simulink model "Ball_and_Plate_MicroLabBox_student_v2019"  (R2019b)
settings: Solver=ode1  StartTime=0.0  StopTime=Inf  FixedStep=0.001  RelTol=1e-3
PostLoadFcn:
  | , if any(exist('dsrtsu_mdlpostloadfcn', 'file') ~= 0), dsrtsu_mdlpostloadfcn('Execute', bdroot); end,
InitFcn:
  | , if any(exist('rtifpga_mdlclblib', 'file') ~= 0), rtifpga_mdlclblib('Init', bdroot); end,
values from neighbouring files (symbols this model uses):
  A_robust = K_robust.A    [Init_workspace.m]    (also in OptimalControlleerSythesisNew.m = K.A)
  B_robust = K_robust.B    [Init_workspace.m]    (also in OptimalControlleerSythesisNew.m = K.B)
  ball_pos_sat = 0.2    [Init_workspace.m]
  ball_vel_sat = 1    [Init_workspace.m]
  Baw_robust = C_robust' / (C_robust*C_robust' + aw_reg*eye(2))    [OptimalControlleerSythesisNew.m]
  C_robust = K_robust.C    [Init_workspace.m]    (also in OptimalControlleerSythesisNew.m = K.C)
  D_robust = K_robust.D    [Init_workspace.m]    (also in OptimalControlleerSythesisNew.m = K.D)
  g = 9.81    [Init_workspace.m]    (also in OptimalControlleerSythesis.m; OptimalControlleerSythesisNew.m; Robustcontroller_angleOutput_Hinf_positionSensitive_center034.m; compute_mpc_params.m)
  K_lqr = dlqr(Ad, Bd, Q_lqr, R_lqr)    [Init_workspace.m]
  Kaw_robust = 0.15    [OptimalControlleerSythesisNew.m]
  path = quintic(-0.0289,3,0,1/fs)    [Init_workspace.m]    (also in Quintic_Time.m = reference_end; Quintic_Velocity.m = reference_end)
  plate_angle_sat = deg2rad(10)    [Init_workspace.m]
  Q_kf = diag([1, 100, 1, 100])    [Init_workspace.m]
  R_kf = diag([0.1, 0.1])    [Init_workspace.m]
  Ts_Outer = 1/50    (= 0.02)    [Init_workspace.m]
  u_max_robust = [ alpha_lim;  beta_lim]    [OptimalControlleerSythesisNew.m]
  u_min_robust = [-alpha_lim; -beta_lim]    [OptimalControlleerSythesisNew.m]
  uA = repmat(uA,[1,P])    [Init_workspace.m]
  uB = repmat(uB,[1,P])    [Init_workspace.m]
  uC = repmat(uC,[1,P])    [Init_workspace.m]
undefined symbols (not defined in the file or in its folder): a_circ, a_square, DiscIntNeverNeededParam, inner_I_sat, r_circ, r_square, Ts_Inner
libraries: simulink x7, rtiemclib x6, rtiethernetlib x3, rti1202lib_dac_class1 x3, slrealtimeutilitieslib x1, mpclib x1
(part 3 of 3)

== system Ball_and_Plate_MicroLabBox_student_v2019/Innerloop_Actuator/Motor_C/Position Measurement ==
  Init : Inport
  AbsPosition : Sum  Inputs=-+-  SaturateOnIntegerOverflow=on
  Constant : Constant  Value=10
  EMC_ENCODER_BL1 : rtiemclib/EMC_ENCODER_BL1  DSProperties=struct('RTI',struct('Version',uint32(2),'BlockType',struct('isSLSource',uint8(1),'isSLSink',uint8(0),'isHWSource',uint8(1),'isHWSink',uint8(0),'isSetup',uint8(0),'isInline',uint8(1),'isNonInline',uint8(0),'isInterrupt',uint8(0),'isChannelwise',uint8(1)),'IOBoardType','DSEMC','UnitType','ENCODER','Identifier','ENCODER','DialogType','ML','BlockSet','RTIEMC','SlaveProcessor','NONE'))  RTIBlockInterface=struct('OutputPortsWidth',int32([1 1 1]),'OutputPortsActive',int32([1 1 0]),'OutputPortsName',{{'Position','Speed',['Index Detected']}},'OutputPortsDataType',{{'SS_DOUBLE','SS_DOUBLE','SS_BOOLEAN'}},'InitLevel',3,'IconTransparency','on','BlockDisplay',{{['EMC Encoder\nUnit: 3\nDIO class: 2\nPort: 1\nChannel: 5'],'center'}},'DialogFcn','rtiemcencodergui','BlockName',struct('Token',{{'EMC_ENCODER_BL1'}}))  RTIBlockParameters=struct('UnitNo',{{3,'OFF',[1 6]}},'DioClassNo',{{2,'OFF',[1 2]}},'PortNo',{{1,'OFF',[1 1]}},'ChannelNo',{{5,'OFF',[1 11]}},'HwSignalPin',{{['DIO1 ch1'],'OFF',[]}},'HwRefPin',{{'GND','OFF',[]}},'EnablePosMeasurement',{{1,'OFF',[0 1]}},'IndexSetMode',{{1,'OFF',[1 3]}},'EnableMinSpeed',{{0,'OFF',[0 1]}},'NumOfLines',{{'1024','OFF',[1 2097152]}},'InitAngleValue',{{'60','OFF',[0 359.99999]}},'IndexAngleValue',{{'0','OFF',[0 359.99999]}},'MinSpeedAngleValue',{{'45','OFF',[0.05 10000]}},'MinPosValue',{{'0','OFF',[-2097152 2097150.75]}},'MaxPosValue',{{'10000','OFF',[-2097151 2097151.75]}},'InitPosValue',{{'0','OFF',[-2097152 2097151.75]}},'IndexPosValue',{{'0','OFF',[-2097152 2097151.75]}},'MinSpeedPosValue',{{'100','OFF',[1 1000000]}},'IndexGateMode',{{0,'OFF',[0 1]}},'EnableNoiseFilter',{{0,'OFF',[0 1]}},'FilterInterval',{{'0','OFF',[0 0.01]}},'IndexDetectedOutPortMode',{{0,'OFF',[0 1]}},'BuildCheckAngleMeasurement',{{0,'OFF',[0 1]}},'BuildCheckAngleIndexMode',{{0,'OFF',[0 1]}},'BuildCheckPosIndexMode',{{0,'OFF',[0 1]}},'BuildCheckAngleMinSpeed',{{0,'OFF',[0 1]}},'BuildCheckPosMinSpeed',{{0,'OFF',[0 1]}},'TLCFileName',{{'rtiemcencoder','OFF',[]}})  RTISFcnParameters=struct('UnitNo','int32','DioClassNo','int32','PortNo','int32','ChannelNo','int32','EnablePosMeasurement','int32','IndexSetMode','int32','IndexDetectedOutPortMode','int32','EnableMinSpeed','int32','NumOfLines','uint32','InitAngleValue','double','IndexAngleValue','double','MinSpeedAngleValue','double','MinPosValue','double','MaxPosValue','double','InitPosValue','double','IndexPosValue','double','MinSpeedPosValue','double','IndexGateMode','int32','EnableNoiseFilter','int32','FilterInterval','double','TLCFileName','char')  RTIBlockParaDefault=struct('UnitNo',1,'DioClassNo',1,'PortNo',1,'ChannelNo',1,'HwSignalPin',['DIO1 ch1'],'HwRefPin','GND','EnablePosMeasurement',0,'IndexSetMode',1,'EnableMinSpeed',0,'NumOfLines',1024,'InitAngleValue',60,'IndexAngleValue',0,'MinSpeedAngleValue',45,'MinPosValue',0,'MaxPosValue',1023.75,'InitPosValue',0,'IndexPosValue',0,'MinSpeedPosValue',100,'IndexGateMode',0,'EnableNoiseFilter',0,'FilterInterval',0,'IndexDetectedOutPortMode',0,'BuildCheckAngleMeasurement',1,'BuildCheckAngleIndexMode',0,'BuildCheckPosIndexMode',0,'BuildCheckAngleMinSpeed',0,'BuildCheckPosMinSpeed',0,'TLCFileName','rtiemcencoder')
      settings: SourceProductName=dSPACE RTI Electric Motor Control Blockset
  EMC_ENCODER_POS_SET_BL1 : rtiemclib/EMC_ENCODER_POS_SET_BL1  DSProperties=struct('RTI',struct('Version',uint32(1),'BlockType',struct('isSLSource',uint8(0),'isSLSink',uint8(1),'isHWSource',uint8(0),'isHWSink',uint8(1),'isSetup',uint8(0),'isInline',uint8(1),'isNonInline',uint8(0),'isInterrupt',uint8(0),'isChannelwise',uint8(1)),'IOBoardType','DSEMC','UnitType','ENCODER','Identifier','ENCODERPOSSET','DialogType','ML','BlockSet','RTIEMC','SlaveProcessor','NONE'))  RTIBlockInterface=struct('InputPortsWidth',int32(1),'InputPortsActive',1,'InputPortsDataType',{{'SS_DOUBLE'}},'InputPortsName',{{'Position'}},'TriggerPort',{{'rising'}},'InitLevel',3,'IconTransparency','on','BlockDisplay',{{['EMC Encoder Position Set\nUnit: 3\nDIO class: 2\nPort: 1\nChannel: 5'],'center'}},'DialogFcn','rtiemcencoderpossetgui','BlockName',struct('Token',{{'EMC_ENCODER_POS_SET_BL1'}}))  RTIBlockParameters=struct('EncoderIdIndex',{{4,'OFF',[1 4]}},'UnitNo',{{3,'OFF',[]}},'DioClassNo',{{2,'OFF',[]}},'PortNo',{{1,'OFF',[]}},'ChannelNo',{{5,'OFF',[]}},'EnablePosMeasurement',{{1,'OFF',[]}},'NumOfLines',{{1024,'OFF',[]}},'TLCFileName',{{'rtiemcencoderposset','OFF',[]}})  RTISFcnParameters=struct('EncoderIdIndex','int32','UnitNo','int32','DioClassNo','int32','PortNo','int32','ChannelNo','int32','EnablePosMeasurement','int32','NumOfLines','int32','TLCFileName','char')  RTIBlockParaDefault=struct('EncoderIdIndex',1,'UnitNo',-1,'DioClassNo',-1,'PortNo',-1,'ChannelNo',-1,'EnablePosMeasurement',0,'NumOfLines',1024,'TLCFileName','rtiemcencoderposset')
      settings: SourceProductName=dSPACE RTI Electric Motor Control Blockset
  Inc2Pos : Gain  Gain=8e-3  SaturateOnIntegerOverflow=on  OutDataTypeStr=Inherit: Same as input  ParamDataTypeStr=Inherit: Same as input
  Initial : Subsystem
  Pos_offset : Constant  Value=0
  ZP : Constant  Value=29
  mm2m : Gain  Gain=0.001
  init_current : Outport  VectorParamsAs1DForOutWhenUnconnected=off
  Position [m] : Outport  Port=2  VectorParamsAs1DForOutWhenUnconnected=off
  wires:
  AbsPosition/1 -> mm2m/1
  Inc2Pos/1 -> Initial/1(Pos), AbsPosition/2
  Initial/2(init_current) -> init_current/1
  mm2m/1 -> Position [m]/1
  EMC_ENCODER_BL1/2 -> Initial/2(DeltaPos)
  ZP/1 -> AbsPosition/1
  Constant/1 -> EMC_ENCODER_POS_SET_BL1/1
  Init/1 -> Initial/3(Init), EMC_ENCODER_POS_SET_BL1/Trigger
  Pos_offset/1 -> AbsPosition/3
  EMC_ENCODER_BL1/1 -> Inc2Pos/1

== system Ball_and_Plate_MicroLabBox_student_v2019/Innerloop_Actuator/Motor_C/motorC ==
  Input : Inport
  I_reset : Inport  Port=2
  Add : Sum
  Dct1lowpass1 : S-Function  FunctionName=dlowpass1  Parameters=f_den, 0.001  SFunctionDeploymentMode=off  EnableBusSupport=off  mask(dctools){f_den=50}
      mask prompts: f_den "Pole [Hz]"
      mask help: This block implements a discrete time 1st order lowpass filter.
      mask Display: disp('DCT 1st order lowpass')
  Dct1lowpass2 : S-Function  Commented=on  FunctionName=dlowpass1  Parameters=f_den, 0.001  SFunctionDeploymentMode=off  EnableBusSupport=off  mask(dctools){f_den=50}
      mask prompts: f_den "Pole [Hz]"
      mask help: This block implements a discrete time 1st order lowpass filter.
      mask Display: disp('DCT 1st order lowpass')
  Dctleadlag1 : S-Function  FunctionName=dleadlag  Parameters=f_num, f_den, 0.001  SFunctionDeploymentMode=off  EnableBusSupport=off  mask(dctools){f_num=7.5, f_den=30}
      mask prompts: f_num "Zero [Hz]"; f_den "Pole [Hz]"
      mask help: This block implements a discrete time leadlag filter.
      mask Display: disp('DCT leadlag')
  Dctleadlag2 : S-Function  Commented=on  FunctionName=dleadlag  Parameters=f_num, f_den, 0.001  SFunctionDeploymentMode=off  EnableBusSupport=off  mask(dctools){f_num=7.5, f_den=45}
      mask prompts: f_num "Zero [Hz]"; f_den "Pole [Hz]"
      mask help: This block implements a discrete time leadlag filter.
      mask Display: disp('DCT leadlag')
  Discrete-Time Integrator : DiscreteIntegrator  gainval=2500  ExternalReset=rising  SampleTime=-1  LimitOutput=on  UpperSaturationLimit=inner_I_sat  LowerSaturationLimit=-inner_I_sat  ICPrevOutput=DiscIntNeverNeededParam  ICPrevScaledInput=DiscIntNeverNeededParam
  Gain1 : Gain  Commented=on  Gain=350  SaturateOnIntegerOverflow=on  OutDataTypeStr=Inherit: Same as input  ParamDataTypeStr=Inherit: Same as input
  Gain2 : Gain  Gain=400  SaturateOnIntegerOverflow=on  OutDataTypeStr=Inherit: Same as input  ParamDataTypeStr=Inherit: Same as input
  Output : Outport
  wires:
  Add/1 -> Output/1
  Dctleadlag1/1 -> Dct1lowpass1/1
  Input/1 -> Gain2/1, Discrete-Time Integrator/1
  Dct1lowpass1/1 -> Add/1
  I_reset/1 -> Discrete-Time Integrator/2
  Gain2/1 -> Dctleadlag1/1
  Discrete-Time Integrator/1 -> Add/2
  Gain1/1 -> Dctleadlag2/1
  Dctleadlag2/1 -> Dct1lowpass2/1

== system Ball_and_Plate_MicroLabBox_student_v2019/RTI Data/RTI Data Store/RTI Data Store ==
  RTI Data Store : Subsystem  mask(RTI_DATA_STORE){}
      mask help:
      | RTI Data Store Block. This block is used by RTI to store internal model dependent data. Deleting this block will result in data loss.
      |
      | NEVER DELETE, COPY, OR MODIFY THIS BLOCK!
      mask Help:
      | RTI Data Store Block. This block is used by RTI to store internal model dependent data. Deleting this block will result in data loss.
      | 
      | NEVER DELETE, COPY, OR MODIFY THIS BLOCK!
      mask Display: text(0.5, 0.5, ' ', 'HorizontalAlignment', 'center');

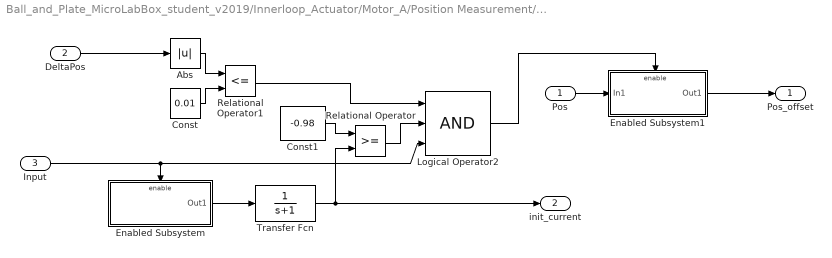
== system Ball_and_Plate_MicroLabBox_student_v2019/Innerloop_Actuator/Motor_A/Position Measurement/Initial ==
  Pos : Inport
  DeltaPos : Inport  Port=2
  Input : Inport  Port=3
  Abs : Abs  SaturateOnIntegerOverflow=on
  Const : Constant  Value=0.01
  Const1 : Constant  Value=-0.98
  Enabled Subsystem : Subsystem  TreatAsAtomicUnit=on
  Enabled Subsystem1 : Subsystem  TreatAsAtomicUnit=on
  Logical Operator2 : Logic  Inputs=3  AllPortsSameDT=off
  Relational Operator : RelationalOperator  RndMeth=Nearest
  Relational Operator1 : RelationalOperator  Operator=<=  RndMeth=Nearest
  Transfer Fcn : TransferFcn  Denominator=[1 1]
  Pos_offset : Outport  VectorParamsAs1DForOutWhenUnconnected=off
  init_current : Outport  Port=2  VectorParamsAs1DForOutWhenUnconnected=off
  wires:
  Enabled Subsystem/1(Out1) -> Transfer Fcn/1
  Transfer Fcn/1 -> Relational Operator/2, init_current/1
  Input/1 -> Enabled Subsystem/Enable, Logical Operator2/3
  Const1/1 -> Relational Operator/1
  Abs/1 -> Relational Operator1/1
  Const/1 -> Relational Operator1/2
  Relational Operator1/1 -> Logical Operator2/1
  Relational Operator/1 -> Logical Operator2/2
  DeltaPos/1 -> Abs/1
  Logical Operator2/1 -> Enabled Subsystem1/Enable
  Pos/1 -> Enabled Subsystem1/1(In1)
  Enabled Subsystem1/1(Out1) -> Pos_offset/1

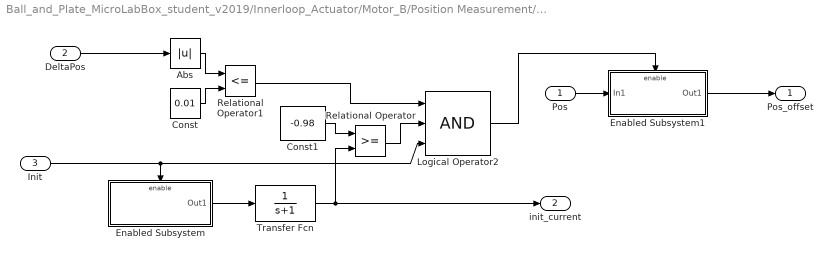
== system Ball_and_Plate_MicroLabBox_student_v2019/Innerloop_Actuator/Motor_B/Position Measurement/Initial ==
  Pos : Inport
  DeltaPos : Inport  Port=2
  Init : Inport  Port=3
  Abs : Abs  SaturateOnIntegerOverflow=on
  Const : Constant  Value=0.01
  Const1 : Constant  Value=-0.98
  Enabled Subsystem : Subsystem  TreatAsAtomicUnit=on
  Enabled Subsystem1 : Subsystem  TreatAsAtomicUnit=on
  Logical Operator2 : Logic  Inputs=3  AllPortsSameDT=off
  Relational Operator : RelationalOperator  RndMeth=Nearest
  Relational Operator1 : RelationalOperator  Operator=<=  RndMeth=Nearest
  Transfer Fcn : TransferFcn  Denominator=[1 1]
  Pos_offset : Outport  VectorParamsAs1DForOutWhenUnconnected=off
  init_current : Outport  Port=2  VectorParamsAs1DForOutWhenUnconnected=off
  wires:
  Enabled Subsystem/1(Out1) -> Transfer Fcn/1
  Transfer Fcn/1 -> Relational Operator/2, init_current/1
  Init/1 -> Enabled Subsystem/Enable, Logical Operator2/3
  Const1/1 -> Relational Operator/1
  Abs/1 -> Relational Operator1/1
  Const/1 -> Relational Operator1/2
  Relational Operator1/1 -> Logical Operator2/1
  Relational Operator/1 -> Logical Operator2/2
  DeltaPos/1 -> Abs/1
  Logical Operator2/1 -> Enabled Subsystem1/Enable
  Pos/1 -> Enabled Subsystem1/1(In1)
  Enabled Subsystem1/1(Out1) -> Pos_offset/1

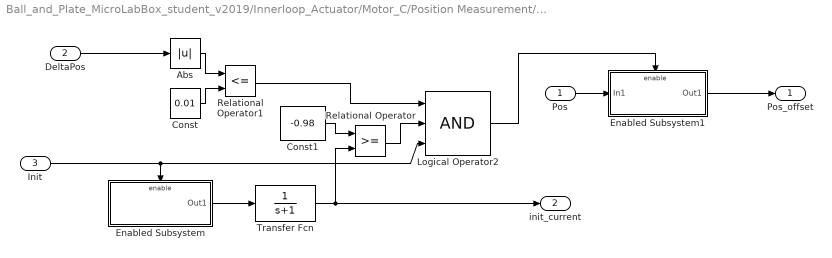
== system Ball_and_Plate_MicroLabBox_student_v2019/Innerloop_Actuator/Motor_C/Position Measurement/Initial ==
  Pos : Inport
  DeltaPos : Inport  Port=2
  Init : Inport  Port=3
  Abs : Abs  SaturateOnIntegerOverflow=on
  Const : Constant  Value=0.01
  Const1 : Constant  Value=-0.98
  Enabled Subsystem : Subsystem  TreatAsAtomicUnit=on
  Enabled Subsystem1 : Subsystem  TreatAsAtomicUnit=on
  Logical Operator2 : Logic  Inputs=3  AllPortsSameDT=off
  Relational Operator : RelationalOperator  RndMeth=Nearest
  Relational Operator1 : RelationalOperator  Operator=<=  RndMeth=Nearest
  Transfer Fcn : TransferFcn  Denominator=[1 1]
  Pos_offset : Outport  VectorParamsAs1DForOutWhenUnconnected=off
  init_current : Outport  Port=2  VectorParamsAs1DForOutWhenUnconnected=off
  wires:
  Enabled Subsystem/1(Out1) -> Transfer Fcn/1
  Transfer Fcn/1 -> Relational Operator/2, init_current/1
  Init/1 -> Enabled Subsystem/Enable, Logical Operator2/3
  Const1/1 -> Relational Operator/1
  Abs/1 -> Relational Operator1/1
  Const/1 -> Relational Operator1/2
  Relational Operator1/1 -> Logical Operator2/1
  Relational Operator/1 -> Logical Operator2/2
  DeltaPos/1 -> Abs/1
  Logical Operator2/1 -> Enabled Subsystem1/Enable
  Pos/1 -> Enabled Subsystem1/1(In1)
  Enabled Subsystem1/1(Out1) -> Pos_offset/1

== system Ball_and_Plate_MicroLabBox_student_v2019/RTI Data/RTI Data Store/RTI Data Store/RTI Data Store ==
  RTI Data Store : Subsystem  mask(RTI_DATA_STORE){}
      mask help:
      | RTI Data Store Block. This block is used by RTI to store internal model dependent data. Deleting this block will result in data loss.
      |
      | NEVER DELETE, COPY, OR MODIFY THIS BLOCK!
      mask Help:
      | RTI Data Store Block. This block is used by RTI to store internal model dependent data. Deleting this block will result in data loss.
      | 
      | NEVER DELETE, COPY, OR MODIFY THIS BLOCK!
      mask Display: text(0.5, 0.5, ' ', 'HorizontalAlignment', 'center');

== system Ball_and_Plate_MicroLabBox_student_v2019/Innerloop_Actuator/Motor_A/Position Measurement/Initial/Enabled Subsystem ==
  Enable : EnablePort  PropagateVarSize=During execution
  Constant : Constant  Value=-1
  Out1 : Outport  OutputWhenDisabled=reset  InitialOutput=[0]  VectorParamsAs1DForOutWhenUnconnected=off
  wires:
  Constant/1 -> Out1/1

== system Ball_and_Plate_MicroLabBox_student_v2019/Innerloop_Actuator/Motor_A/Position Measurement/Initial/Enabled Subsystem1 ==
  In1 : Inport
  Enable : EnablePort  PropagateVarSize=During execution
  Out1 : Outport  InitialOutput=[0]  VectorParamsAs1DForOutWhenUnconnected=off
  wires:
  In1/1 -> Out1/1

== system Ball_and_Plate_MicroLabBox_student_v2019/Innerloop_Actuator/Motor_B/Position Measurement/Initial/Enabled Subsystem ==
  Enable : EnablePort  PropagateVarSize=During execution
  Constant : Constant  Value=-1
  Out1 : Outport  OutputWhenDisabled=reset  InitialOutput=[0]  VectorParamsAs1DForOutWhenUnconnected=off
  wires:
  Constant/1 -> Out1/1

== system Ball_and_Plate_MicroLabBox_student_v2019/Innerloop_Actuator/Motor_B/Position Measurement/Initial/Enabled Subsystem1 ==
  In1 : Inport
  Enable : EnablePort  PropagateVarSize=During execution
  Out1 : Outport  InitialOutput=[0]  VectorParamsAs1DForOutWhenUnconnected=off
  wires:
  In1/1 -> Out1/1

== system Ball_and_Plate_MicroLabBox_student_v2019/Innerloop_Actuator/Motor_C/Position Measurement/Initial/Enabled Subsystem ==
  Enable : EnablePort  PropagateVarSize=During execution
  Constant : Constant  Value=-1
  Out1 : Outport  OutputWhenDisabled=reset  InitialOutput=[0]  VectorParamsAs1DForOutWhenUnconnected=off
  wires:
  Constant/1 -> Out1/1

== system Ball_and_Plate_MicroLabBox_student_v2019/Innerloop_Actuator/Motor_C/Position Measurement/Initial/Enabled Subsystem1 ==
  In1 : Inport
  Enable : EnablePort  PropagateVarSize=During execution
  Out1 : Outport  InitialOutput=[0]  VectorParamsAs1DForOutWhenUnconnected=off
  wires:
  In1/1 -> Out1/1

== system Ball_and_Plate_MicroLabBox_student_v2019/RTI Data/RTI Data Store/RTI Data Store/RTI Data Store/RTI Data Store ==

== matlab function Ball_and_Plate_MicroLabBox_student_v2019/Subsystem/MATLAB Function1 ==
  settings: updateMethod=DISCRETE
  data: e_x input; u_cmd output; ev_x input; e_y input; ev_y input; reset input; Arob input; Brob input; Crob input; Drob input; Baw input; Kaw input; umin input; umax input; u_raw output; u_box output; sat_flag output; xK_norm output
function [u_cmd, u_raw, u_box, sat_flag, xK_norm] = Hinf( ...
    e_x, ev_x, e_y, ev_y, ...
    reset, ...
    Arob, Brob, Crob, Drob, ...
    Baw, Kaw, ...
    umin, umax)
%#codegen
%
% Hinf controller with:
%   1) hard angle saturation
%   2) command rate limiting
%   3) anti-windup based on the ACTUAL command sent to the plant
%
% Inputs:
%   e_x, ev_x, e_y, ev_y = [r_x-x; -xdot; r_z-z; -zdot]
%   reset                = 1 when outer loop disabled
%
% Outputs:
%   u_cmd = final command to plant / AngleToPos
%   u_raw = unconstrained Hinf output
%   u_box = amplitude-saturated Hinf output before rate limit

persistent xK u_prev initialized

nK = size(Arob,1);

if isempty(initialized)
    xK = zeros(nK,1);
    u_prev = zeros(2,1);
    initialized = true;
end

u_raw = zeros(2,1);
u_box = zeros(2,1);
u_cmd = zeros(2,1);
sat_flag = false;
xK_norm = 0;

% Reset controller state while outer loop is off
if reset ~= 0
    xK = zeros(nK,1);
    u_prev = zeros(2,1);
    return;
end

%% Inputs to Hinf controller

yK = [e_x; ev_x; e_y; ev_y];

u_min = [umin(1); umin(2)];
u_max = [umax(1); umax(2)];

%% Raw Hinf command

u_raw = Crob*xK + Drob*yK;

%% Hard amplitude saturation

u_box = min(max(u_raw, u_min), u_max);

%% Rate limit the command sent to the plant

Ts_outer = 0.02;              % Hinf sample time [s]
maxRate  = deg2rad(20.0);    % [rad/s]

du_max = maxRate * Ts_outer;

du = u_box - u_prev;

du_limited = min(max(du, [-du_max; -du_max]), [du_max; du_max]);

u_cmd = u_prev + du_limited;

% Final safety saturation
u_cmd = min(max(u_cmd, u_min), u_max);

%% Anti-windup
% Use the actual plant command, not only the amplitude-saturated command.

du_aw = u_cmd - u_raw;

x_nom = Arob*xK + Brob*yK;
x_next = x_nom + Kaw*(Baw*du_aw);

% Numerical guard
if any(~isfinite(x_next)) || norm(x_next) > 1e8
    x_next = zeros(nK,1);
    u_cmd = zeros(2,1);
end

xK = x_next;
u_prev = u_cmd;

sat_flag = any(abs(u_cmd - u_raw) > 1e-10);
xK_norm = norm(xK);
end

== matlab function Ball_and_Plate_MicroLabBox_student_v2019/Innerloop_Actuator/Motor_A/MATLAB Function ==
  data: e input; u output; reset_integrator input
function u = fcn(e, reset_integrator)
% You need to fill here

u = 0;

== matlab function Ball_and_Plate_MicroLabBox_student_v2019/Innerloop_Actuator/Motor_B/MATLAB Function1 ==
  data: e input; u output; reset_integrator input
function u = fcn(e, reset_integrator)
% You need to fill here

u = 0;

== matlab function Ball_and_Plate_MicroLabBox_student_v2019/Innerloop_Actuator/Motor_A/Multisine/MATLAB Function ==
  data: enable input; u input; y output
function y = Multisine_id(enable, u)

persistent index previous_enable

% Initialize
if isempty(index)
    index = 1;
end

if isempty(previous_enable)
    previous_enable = 0;
end

N = length(u);

% Detect rising edge (re-enable)
if enable && ~previous_enable
    index = 1;
end

% Output logic
if enable

    % If still inside signal → output sample
    if index <= N
        y = u(index);
        index = index + 1;

    else
        % Signal finished → output zero
        y = 0;
    end

else
    % Disabled → output zero
    y = 0;
end

previous_enable = enable;

== matlab function Ball_and_Plate_MicroLabBox_student_v2019/Innerloop_Actuator/Motor_B/Multisine/MATLAB Function ==
  data: enable input; u input; y output
function y = Multisine_id(enable, u)

persistent index previous_enable

% Initialize
if isempty(index)
    index = 1;
end

if isempty(previous_enable)
    previous_enable = 0;
end

N = length(u);

% Detect rising edge (re-enable)
if enable && ~previous_enable
    index = 1;
end

% Output logic
if enable

    % If still inside signal → output sample
    if index <= N
        y = u(index);
        index = index + 1;

    else
        % Signal finished → output zero
        y = 0;
    end

else
    % Disabled → output zero
    y = 0;
end

previous_enable = enable;

== matlab function Ball_and_Plate_MicroLabBox_student_v2019/Innerloop_Actuator/Motor_C/Multisine/MATLAB Function ==
  data: enable input; u input; y output
function y = Multisine_id(enable, u)

persistent index previous_enable

% Initialize
if isempty(index)
    index = 1;
end

if isempty(previous_enable)
    previous_enable = 0;
end

N = length(u);

% Detect rising edge (re-enable)
if enable && ~previous_enable
    index = 1;
end

% Output logic
if enable

    % If still inside signal → output sample
    if index <= N
        y = u(index);
        index = index + 1;

    else
        % Signal finished → output zero
        y = 0;
    end

else
    % Disabled → output zero
    y = 0;
end

previous_enable = enable;

== matlab function Ball_and_Plate_MicroLabBox_student_v2019/coordinates_ball ==
  data: x_2_pixels input; x_2 output; y_2_pixels input; y_2 output; theta_1 input; theta_2 input
function [x_2, y_2] = fcn(x_2_pixels, y_2_pixels, theta_1, theta_2)
    %A01_fun
    %    OUT1 = A01_fun(THETA_1,THETA_2)
    
    %    This function was generated by the Symbolic Math Toolbox version 9.3.
    %    22-May-2025 12:09:11
    y_offset = 242.82;
    x_offset = 295.83;
    conversion_factor = 1120.25;
%     ball_radius = 20e-3;%mm
    x_2_e0 = (double(x_2_pixels)-x_offset)/conversion_factor;
    y_2_e0 = (double(y_2_pixels)-y_offset)/conversion_factor;
    t2 = cos(theta_1);
    t3 = cos(theta_2);
    t4 = sin(theta_1);
    t5 = sin(theta_2);
    out1 = reshape([t3,t4.*t5,-t2.*t5,0.0,t2,t4,t5,-t3.*t4,t2.*t3],[3,3]);
%     temp = double([x_2_e0, y_2_e0, -ball_radius])*double(out1);
    x_2 = x_2_e0;%temp(1);
    y_2 = y_2_e0;%temp(2);
end

== matlab function Ball_and_Plate_MicroLabBox_student_v2019/Innerloop_Actuator/Motor_C/Multisine1/MATLAB Function ==
  data: enable input; u input; y output
function y = Multisine_id(enable, u)

persistent index previous_enable

% Initialize
if isempty(index)
    index = 1;
end

if isempty(previous_enable)
    previous_enable = 0;
end

N = length(u);

% Detect rising edge (re-enable)
if enable && ~previous_enable
    index = 1;
end

% Output logic
if enable

    % If still inside signal → output sample
    if index <= N
        y = u(index);
        index = index + 1;

    else
        % Signal finished → output zero
        y = 0;
    end

else
    % Disabled → output zero
    y = 0;
end

previous_enable = enable;

== matlab function Ball_and_Plate_MicroLabBox_student_v2019/Innerloop_Actuator/Motor_B/Init_motion/MATLAB Function1 ==
  data: reference_end input; path output; end_time input; Ts input; measured_position input
function path = Quintic_Polynomial_Trajectory_Time(reference_end, end_time, Ts, measured_position)
%% Quintic_Polynomial_Trajectory(reference_end, average_velocity)
% This function outputs a quintic polynomial trajectory over time in 
% Simulink given the end reference and average velocity. The starting 
% velocity and acceleration are set to zero.
%
% Input Arguments
% reference_end = desired end position of the trajectory
% end_time = end time of trajectory; for every new input 
% trajectory starts at time 0 and ends at end_time
% measured_position = current position of the robot arm
%
% Output Arguments
% path = path of the trajectory over time
%
% Quinten Swaan 17-08-2022
%
% Control Systems Technology group
% Departement of Mechanical Engineering
% Eindhoven University of Technology


persistent previous_value_reference_start previous_value_reference_end ...
    path_array index 

if isempty(previous_value_reference_start)
    previous_value_reference_start = 0;
end

if isempty(previous_value_reference_end)
    previous_value_reference_end = 0;
end

if isempty(path_array)
    path_array = zeros(1,1);
end

if isempty(index)
    index = 1;
end


% Obtain new trajectory if a new end reference is given
if previous_value_reference_end ~= reference_end
    t0 = 0;                                 %Starting time
    q0 = previous_value_reference_start;    %Starting position
    v0 = 0;                                 %Starting velocity
    ac0 = 0;                                %Starting acceleration
    tf = end_time;                          %End time
    qf = reference_end;                     %End position
    vf = 0;                                 %End velocity
    acf = 0;                                %End acceleration

    M = [1 t0 t0^2 t0^3 t0^4 t0^5;
    0 1 2*t0 3*t0^2 4*t0^3 5*t0^4;
    0 0 2 6*t0 12*t0^2 20*t0^3;
    1 tf tf^2 tf^3 tf^4 tf^5;
    0 1 2*tf 3*tf^2 4*tf^3 5*tf^4;
    0 0 2 6*tf 12*tf^2 20*tf^3];

    b = [q0; v0; ac0; qf; vf; acf];

    x = M \ b;

    t = t0:Ts:tf;

    path_array = x(1) + x(2).*t + x(3).*t.^2 + x(4).*t.^3 + +x(5).*t.^4 + x(6).*t.^5;

    index = 1;
    reference_current = path_array(index);

% Output the reference per timestep
else
    if index < length(path_array)
        index = index + 1;
    end
    reference_current = path_array(index);
end

previous_value_reference_end = reference_end;
previous_value_reference_start = measured_position;

path = reference_current;

== matlab function Ball_and_Plate_MicroLabBox_student_v2019/Innerloop_Actuator/Motor_B/Init_motion/MATLAB Function2 ==
  data: y input; path output; start input; init_value input; current_pos input
function path = init_motion(y, start, init_value, current_pos)

if start > 0.5
    path = init_value;
elseif start < 0.5
    path = y;
else 
    path = 0;
end

== matlab function Ball_and_Plate_MicroLabBox_student_v2019/circ_ref_player  ==
  data: r input; rsample output; a input; enable input; asample output; rpreview output
function [rsample, asample, rpreview] = ref_player(r, a, enable)
%#codegen
Npreview = 25; % number of samples preview for MPC

% Persistent variable to track the current sample index
persistent idx_ref;

% Initialize the index on the very first time step
if isempty(idx_ref)
    idx_ref = 1;
end

% Determine the total number of offline samples available
N_total = size(r, 2);

% Preallocate outputs for code generation stability
rsample = zeros(4, 1);
asample = zeros(2, 1);
% CHANGED: 25 rows (time steps), 4 columns (states)
rpreview = zeros(Npreview, 4); 

% --- Trajectory Generation Logic ---
if enable == 1
    % 1. Extract the current sample
    if idx_ref <= N_total
        rsample = r(:, idx_ref);
        asample = a(:, idx_ref);
    else
        % Hold the final sample if the trajectory ends but enable stays 1
        rsample = r(:, N_total);
        asample = a(:, N_total);
    end
    
    % 2. Extract the next Npreview samples for MPC
    for i = 1:Npreview
        preview_idx = idx_ref + i; 
        
        if preview_idx <= N_total
            % CHANGED: Assign transposed column [1x4] into row i
            rpreview(i, :) = r(:, preview_idx)'; 
        else
            % Zero-order hold: Pad with the last available reference state 
            rpreview(i, :) = r(:, N_total)';
        end
    end
    
    % 3. Advance the index for the next sample time (Ts)
    if idx_ref <= N_total
        idx_ref = idx_ref + 1;
    end
else
    % --- Reset / Idle State (enable == 0) ---
    % Keep index reset to the first sample
    idx_ref = 1; 
    
    % Output the initial conditions while waiting
    rsample = r(:, 1);
    asample = a(:, 1);
    
    % Provide a static look-ahead from the starting point
    for i = 1:Npreview
        if (1 + i) <= N_total
            % CHANGED: Transpose required here too
            rpreview(i, :) = r(:, 1 + i)';
        else
            rpreview(i, :) = r(:, N_total)';
        end
    end
end

== matlab function Ball_and_Plate_MicroLabBox_student_v2019/square_ref_player  ==
  data: r input; rsample output; a input; enable input; asample output; rpreview output
function [rsample, asample, rpreview] = ref_player(r, a, enable)
%#codegen
Npreview = 25; % number of samples preview for MPC

% Persistent variable to track the current sample index
persistent idx_ref;

% Initialize the index on the very first time step
if isempty(idx_ref)
    idx_ref = 1;
end

% Determine the total number of offline samples available
N_total = size(r, 2);

% Preallocate outputs for code generation stability
rsample = zeros(4, 1);
asample = zeros(2, 1);
% CHANGED: 25 rows (time steps), 4 columns (states)
rpreview = zeros(Npreview, 4); 

% --- Trajectory Generation Logic ---
if enable == 1
    % 1. Extract the current sample
    if idx_ref <= N_total
        rsample = r(:, idx_ref);
        asample = a(:, idx_ref);
    else
        % Hold the final sample if the trajectory ends but enable stays 1
        rsample = r(:, N_total);
        asample = a(:, N_total);
    end
    
    % 2. Extract the next Npreview samples for MPC
    for i = 1:Npreview
        preview_idx = idx_ref + i; 
        
        if preview_idx <= N_total
            % CHANGED: Assign transposed column [1x4] into row i
            rpreview(i, :) = r(:, preview_idx)'; 
        else
            % Zero-order hold: Pad with the last available reference state 
            rpreview(i, :) = r(:, N_total)';
        end
    end
    
    % 3. Advance the index for the next sample time (Ts)
    if idx_ref <= N_total
        idx_ref = idx_ref + 1;
    end
else
    % --- Reset / Idle State (enable == 0) ---
    % Keep index reset to the first sample
    idx_ref = 1; 
    
    % Output the initial conditions while waiting
    rsample = r(:, 1);
    asample = a(:, 1);
    
    % Provide a static look-ahead from the starting point
    for i = 1:Npreview
        if (1 + i) <= N_total
            % CHANGED: Transpose required here too
            rpreview(i, :) = r(:, 1 + i)';
        else
            rpreview(i, :) = r(:, N_total)';
        end
    end
end

== matlab function Ball_and_Plate_MicroLabBox_student_v2019/Innerloop_Actuator/Motor_B/Init_motion/MATLAB Function ==
  data: enable input; u input; y output
function y = init_motion(enable, u)

persistent index previous_enable

% Initialize
if isempty(index)
    index = 1;
end

if isempty(previous_enable)
    previous_enable = 0;
end

N = length(u);

% Detect rising edge (re-enable)
if enable && ~previous_enable
    index = 1;
end

% Output logic
if enable

    % If still inside signal → output sample
    if index <= N
        y = u(index);
        index = index + 1;

    else
        % Signal finished → output zero
        y = 0;
    end

else
    % Disabled → output zero
    y = -0.0289;
end

previous_enable = enable;

== matlab function Ball_and_Plate_MicroLabBox_student_v2019/Innerloop_Actuator/AngleToPos  ==
  data: alpha input; pos1 output; beta input; psi input; pos2 output; pos3 output
function [pos1, pos2, pos3] = angleToPos(alpha, beta, psi)
    % Returns the actuator positions required to reach the desired angle
    % note: the position is absolute in the global frame

    % Physical Constants
    r = 0.17;           % Joint radius (m)
    T = [0; 0; 0.32];  % Resting height vector (m)
    
    % Joint positions on base and plate (equilateral triangle)
    % These match the definitions in your posToAngle function
    theta = [0, deg2rad(240), deg2rad(120)];
    B = [r*cos(theta); r*sin(theta); zeros(1,3)]; % Base joints (b_i)
    P = [r*cos(theta); r*sin(theta); zeros(1,3)]; % Plate joints (p_i)
    
    % Rotation Matrices (Yaw-Pitch-Roll order)
    Rz = [cos(psi) -sin(psi) 0; sin(psi) cos(psi) 0; 0 0 1];
    Ry = [cos(beta) 0 sin(beta); 0 1 0; -sin(beta) 0 cos(beta)];
    Rx = [1 0 0; 0 cos(alpha) -sin(alpha); 0 sin(alpha) cos(alpha)];
    R_BtoP = Rz * Ry * Rx; 
    
    % Compute absolute position for each motor
    % Motor 1
    l1_vec = T + (R_BtoP * P(:,1)) - B(:,1);
    pos1 = norm(l1_vec);
    
    % Motor 2
    l2_vec = T + (R_BtoP * P(:,2)) - B(:,2);
    pos2 = norm(l2_vec);
    
    % Motor 3
    l3_vec = T + (R_BtoP * P(:,3)) - B(:,3);
    pos3 = norm(l3_vec);
end

== matlab function Ball_and_Plate_MicroLabBox_student_v2019/Innerloop_Actuator/Motor_A/MATLAB Function1 ==
  data: reference_end input; path output; end_time input; Ts input; measured_position input
function path = Quintic_Time(reference_end, end_time, Ts, measured_position)
% QUINTIC_POLYNOMIAL_TRAJECTORY_TIME
% Calculated analytically per step to be compatible with dSPACE/Control Desk.

% Persistent variables to store coefficients and the "internal clock"
persistent coeffs t_elapsed prev_ref_end tf_internal
if isempty(coeffs)
    coeffs = zeros(6, 1); % a0, a1, a2, a3, a4, a5
end
if isempty(t_elapsed)
    t_elapsed = 0;
end
if isempty(prev_ref_end)
    prev_ref_end = reference_end;
end
if isempty(tf_internal)
    tf_internal = 0;
end

% Check if a new trajectory is requested
if reference_end ~= prev_ref_end
    % Reset timer
    t_elapsed = 0;
    tf_internal = end_time;
    
    % Boundary conditions
    q0 = prev_ref_end; 
    qf = reference_end;
    v0 = 0; vf = 0;
    ac0 = 0; acf = 0;
    
    % Solver for t0 = 0
    % We solve the system: M * coeffs = b
    % Using tf_internal instead of end_time to ensure consistency during the run
    T = tf_internal;
    M = [1, 0, 0,  0,    0,    0;
         0, 1, 0,  0,    0,    0;
         0, 0, 2,  0,    0,    0;
         1, T, T^2, T^3,  T^4,  T^5;
         0, 1, 2*T, 3*T^2, 4*T^3, 5*T^4;
         0, 0, 2,   6*T,   12*T^2, 20*T^3];
     
    b = [q0; v0; ac0; qf; vf; acf];
    
    % Calculate coefficients (Matrix is small 6x6, so this is fast)
    coeffs = M \ b;
end

% Calculate current reference based on elapsed time
t = t_elapsed;

if t <= tf_internal
    % Quintic Equation: path = a0 + a1*t + a2*t^2 + a3*t^3 + a4*t^4 + a5*t^5
    path = coeffs(1) + coeffs(2)*t + coeffs(3)*t^2 + coeffs(4)*t^3 + coeffs(5)*t^4 + coeffs(6)*t^5;
    
    % Increment time for the next step
    t_elapsed = t_elapsed + Ts;
else
    % Hold the final position once trajectory is finished
    path = reference_end;
end

% Update memory for next iteration
prev_ref_end = reference_end;

end

== matlab function Ball_and_Plate_MicroLabBox_student_v2019/Innerloop_Actuator/Motor_B/MATLAB Function2 ==
  data: reference_end input; path output; end_time input; Ts input; measured_position input
function path = Quintic_Time(reference_end, end_time, Ts, measured_position)
% QUINTIC_POLYNOMIAL_TRAJECTORY_TIME
% Calculated analytically per step to be compatible with dSPACE/Control Desk.

% Persistent variables to store coefficients and the "internal clock"
persistent coeffs t_elapsed prev_ref_end tf_internal
if isempty(coeffs)
    coeffs = zeros(6, 1); % a0, a1, a2, a3, a4, a5
end
if isempty(t_elapsed)
    t_elapsed = 0;
end
if isempty(prev_ref_end)
    prev_ref_end = reference_end;
end
if isempty(tf_internal)
    tf_internal = 0;
end

% Check if a new trajectory is requested
if reference_end ~= prev_ref_end
    % Reset timer
    t_elapsed = 0;
    tf_internal = end_time;
    
    % Boundary conditions
    q0 = prev_ref_end; 
    qf = reference_end;
    v0 = 0; vf = 0;
    ac0 = 0; acf = 0;
    
    % Solver for t0 = 0
    % We solve the system: M * coeffs = b
    % Using tf_internal instead of end_time to ensure consistency during the run
    T = tf_internal;
    M = [1, 0, 0,  0,    0,    0;
         0, 1, 0,  0,    0,    0;
         0, 0, 2,  0,    0,    0;
         1, T, T^2, T^3,  T^4,  T^5;
         0, 1, 2*T, 3*T^2, 4*T^3, 5*T^4;
         0, 0, 2,   6*T,   12*T^2, 20*T^3];
     
    b = [q0; v0; ac0; qf; vf; acf];
    
    % Calculate coefficients (Matrix is small 6x6, so this is fast)
    coeffs = M \ b;
end

% Calculate current reference based on elapsed time
t = t_elapsed;

if t <= tf_internal
    % Quintic Equation: path = a0 + a1*t + a2*t^2 + a3*t^3 + a4*t^4 + a5*t^5
    path = coeffs(1) + coeffs(2)*t + coeffs(3)*t^2 + coeffs(4)*t^3 + coeffs(5)*t^4 + coeffs(6)*t^5;
    
    % Increment time for the next step
    t_elapsed = t_elapsed + Ts;
else
    % Hold the final position once trajectory is finished
    path = reference_end;
end

% Update memory for next iteration
prev_ref_end = reference_end;

end

== matlab function Ball_and_Plate_MicroLabBox_student_v2019/Innerloop_Actuator/Motor_C/MATLAB Function1 ==
  data: reference_end input; path output; end_time input; Ts input; measured_position input
function path = Quintic_Time(reference_end, end_time, Ts, measured_position)
% QUINTIC_POLYNOMIAL_TRAJECTORY_TIME
% Calculated analytically per step to be compatible with dSPACE/Control Desk.

% Persistent variables to store coefficients and the "internal clock"
persistent coeffs t_elapsed prev_ref_end tf_internal
if isempty(coeffs)
    coeffs = zeros(6, 1); % a0, a1, a2, a3, a4, a5
end
if isempty(t_elapsed)
    t_elapsed = 0;
end
if isempty(prev_ref_end)
    prev_ref_end = reference_end;
end
if isempty(tf_internal)
    tf_internal = 0;
end

% Check if a new trajectory is requested
if reference_end ~= prev_ref_end
    % Reset timer
    t_elapsed = 0;
    tf_internal = end_time;
    
    % Boundary conditions
    q0 = prev_ref_end; 
    qf = reference_end;
    v0 = 0; vf = 0;
    ac0 = 0; acf = 0;
    
    % Solver for t0 = 0
    % We solve the system: M * coeffs = b
    % Using tf_internal instead of end_time to ensure consistency during the run
    T = tf_internal;
    M = [1, 0, 0,  0,    0,    0;
         0, 1, 0,  0,    0,    0;
         0, 0, 2,  0,    0,    0;
         1, T, T^2, T^3,  T^4,  T^5;
         0, 1, 2*T, 3*T^2, 4*T^3, 5*T^4;
         0, 0, 2,   6*T,   12*T^2, 20*T^3];
     
    b = [q0; v0; ac0; qf; vf; acf];
    
    % Calculate coefficients (Matrix is small 6x6, so this is fast)
    coeffs = M \ b;
end

% Calculate current reference based on elapsed time
t = t_elapsed;

if t <= tf_internal
    % Quintic Equation: path = a0 + a1*t + a2*t^2 + a3*t^3 + a4*t^4 + a5*t^5
    path = coeffs(1) + coeffs(2)*t + coeffs(3)*t^2 + coeffs(4)*t^3 + coeffs(5)*t^4 + coeffs(6)*t^5;
    
    % Increment time for the next step
    t_elapsed = t_elapsed + Ts;
else
    % Hold the final position once trajectory is finished
    path = reference_end;
end

% Update memory for next iteration
prev_ref_end = reference_end;

end

== matlab function Ball_and_Plate_MicroLabBox_student_v2019/Ethernet communication/MATLAB Function ==
  data: x output; u input; y output; z output; flag output
function [x,y,z,flag] = fcn(u)

 x = double(typecast(uint8(u(1:4)), 'single'));
 y = double(typecast(uint8(u(5:8)), 'single'));
 z = double(typecast(uint8(u(9:12)), 'single'));
 
 flag = double(u(13));

%     x = double(u(1)) + 256*double(u(2));
%     y = double(u(5)) + 256*double(u(6));
%     z = double(u(9)) + 256*double(u(10));
%     flag = u(11);
%     
%     if x > 32767
%         x = x-65536;
%     end
%     if y > 32767
%         y = y-65536;
%     end
%     if z > 32767
%         z = z-65536;
%     end
end

== matlab function Ball_and_Plate_MicroLabBox_student_v2019/Innerloop_Actuator/PosToAngle  ==
  data: pos1 input; alpha output; pos2 input; pos3 input; beta output; psi output
function [alpha, beta, psi] = posToAngle(pos1, pos2, pos3)
    % Returns the angles resulting from the given position
    % note: the position should be relative from the actuators midpoint in the global frame

    % Physical Constants
    r = 0.17;                 % Radius to joints (m)
    T = 0.322;                % Resting height (m)
    theta = deg2rad(120);     % angle between bases (rad)

    % Reconstruction of the Plate Unit Vectors 
    % We find where the joints are in the world frame by using the inputs
    % If pos = 0.322, the joints are exactly T_height above the base.
    P1_global = [r; 0; T + pos1];
    P2_global = [r*cos(theta); r*sin(theta); T + pos2];
    P3_global = [r*cos(theta); -r*sin(theta); T + pos3];

    % Find the center of the tilted plate
    % The average of the three joint positions gives the center of the motion plate
    center = (P1_global + P2_global + P3_global) / 3;

    % Vectors from the plate center to the joints
    % This isolates the tilt of the plate surface
    v1 = P1_global - center;
    v2 = P2_global - center;
    v3 = P3_global - center;

    % Compute Unit Vectors
    uX = v1 / norm(v1);             % Plate X-axis
    u_temp = cross(uX, v3);         % Temporary vector to find normal
    uZ = u_temp / norm(u_temp);     % Plate Z-axis (Normal)
    uY = cross(uZ, uX);             % Plate Y-axis

    % Extract Tait-Bryan Angles
    beta = asin(-uX(3));                            
    alpha = asin(uY(3) / sqrt(1 - uX(3)^2));       
    psi = asin(uX(2) / sqrt(1 - uX(3)^2));
end

== matlab function Ball_and_Plate_MicroLabBox_student_v2019/MATLAB Function ==
  settings: updateMethod=DISCRETE
  data: y_meas input; u input; x_est output; valid_frame input; Qkf input; Rkf input; Ts input
function x_est = intermittent_kalman(y_meas, u, valid_frame, Qkf, Rkf, Ts)
    
    g = 9.81;
    Ad = [1, Ts, 0,0;
        0, 1, 0, 0;
        0, 0, 1, Ts;
        0, 0, 0, 1];

    Bd = [5/14 * g * Ts^2, 0;
        5/7 * g * Ts, 0;
        0, 5/14 * g * Ts^2;
        0, 5/7 * g * Ts];
    
    Cd = [1 0 0 0;
        0 0 1 0];


    % Persistent variables keep their state between sample steps
    persistent x_hat P
    
    % Initialization on the very first time step
    if isempty(x_hat)
        x_hat = zeros(4,1);
        P = eye(4) * 0.1;
    end
    
    % 1. Prediction Step (Always executes)
    x_pred = Ad * x_hat + Bd * u;
    P_pred = Ad * P * Ad' + Qkf;
    
    % 2. Correction Step (Conditional)
    if valid_frame > 0.5
        % Frame is valid: Run normal Kalman Correction
        S = Cd * P_pred * Cd' + Rkf;
        K = P_pred * Cd' / S; % Equivalent to P_pred * Cd' * inv(S)
        
        x_hat = x_pred + K * (y_meas - Cd * x_pred);
        P = (eye(4) - K * Cd) * P_pred;
    else
        % Frame was dropped: Skip correction, trust physics prediction
        x_hat =x_pred;
        P = P_pred;
    end
    
    % Output the current state estimate
    x_est = x_hat;
end

== matlab function Ball_and_Plate_MicroLabBox_student_v2019/MATLAB Function3 ==
  data: R input; r output; omega input; Ts input; enable input; a output
function [r,a] = Circle_Reference_spiral(R, omega, Ts, enable)
% CIRCLE_REFERENCE Generates [x; xdot; y; ydot] for a spiral-in/spiral-out trajectory.

% Persistent variables to track phase and the dynamic radius
persistent theta current_R

% Initialize persistent variables on the very first run
if isempty(theta)
    theta = 0;
end
if isempty(current_R)
    current_R = 0; % Start at the origin (0,0)
end

% Define how long you want the spiral transition to take (in seconds)
T_ramp = 5.0; 
R_rate = R / T_ramp; % Radial speed (units per second)

% Determine target radius based on the reset flag
if enable
    R_target = R;  % Spiral inward to origin
else
    R_target = 0;  % Spiral outward to full circle
end

% Smoothly update the current radius and compute dR (radial velocity)
if current_R < R_target
    dR = R_rate;
    current_R = current_R + dR * Ts;
    if current_R > R_target
        current_R = R_target;
        dR = 0;
    end
elseif current_R > R_target
    dR = -R_rate;
    current_R = current_R + dR * Ts;
    if current_R < R_target
        current_R = R_target;
        dR = 0;
    end
else
    dR = 0; % Radius is at target, no radial velocity
end

% Compute current positions and velocities
% Note: Velocities now include the dR component for perfect kinematic accuracy!
x     = current_R * cos(theta);
x_dot = dR * cos(theta) - current_R * omega * sin(theta);

y     = current_R * sin(theta);
y_dot = dR * sin(theta) + current_R * omega * cos(theta);

x_ddot = -2*dR*omega*sin(theta) - current_R*omega^2*cos(theta);
y_ddot = -2*dR*omega*cos(theta) - current_R*omega^2*sin(theta);

r = [x; x_dot; y; y_dot];

a = [x_ddot; y_ddot];

% Integrate the phase for the next time step
next_theta = theta + omega * Ts;

% Wrap theta to [0, 2*pi] to protect numerical precision
theta = mod(next_theta, 2*pi);
end
